simulink model "ADCS2018_Simulink_Full"  (R2018a)
settings: Solver=FixedStepAuto  StartTime=0.0  StopTime=tfinal  FixedStep=ss  RelTol=1e-3  EnableMultiTasking=on
values from neighbouring files (symbols this model uses):
  a1 = -9/11    (= -0.818181818182)    [orbitParameters.m]
  b0 = 2/11    (= 0.181818181818)    [orbitParameters.m]
  b1 = -2/11    (= -0.181818181818)    [orbitParameters.m]
  cr = 1    [orbitParameters.m]
  I = 10^-6*[29290.7 53.8 0.5; 53.8 28639.4 0; 0.5 0 5490.1]    [orbitParameters.m]
  Iw = Hw * 180 / (8000*pi)    [orbitParameters.m]
  Kd = 3.68819*1e-4*0.1/8e-11    (= 461023.75)    [orbitParameters.m]
  kd = 2e-2*min(diag(I))*0.2/3e-9    [orbitParameters.m]
  kep_init = [ semimajoraxis ... (first row only)    [orbitParameters.m]
  Kp = 3.29838*1e-8*0.1/1e-12    (= 3298.38)    [orbitParameters.m]
  mc_max = 0.2    [orbitParameters.m]
  mr = [0.001; -0.001; 0.005]    [orbitParameters.m]
  mr_max = 0.2    [orbitParameters.m]
  omega_o = sqrt(mu/abs(semimajoraxis)^3)    [orbitParameters.m]
  Pitch = 90    [orbitParameters.m]
  Roll = 0    [orbitParameters.m]
  Rx = 30    [orbitParameters.m]
  Ry = 30    [orbitParameters.m]
  Rz = 83    [orbitParameters.m]
  tme_init = [2018 06 07 16 15 0]    [orbitParameters.m]
  vc_max = 5    [orbitParameters.m]
  vr_max = 2.5    [orbitParameters.m]
  wx = 30    [orbitParameters.m]
  wy = 0    [orbitParameters.m]
  wz = 0    [orbitParameters.m]
  Yaw = 0    [orbitParameters.m]
undefined symbols (not defined in the file or in its folder): GHemb, GHsim, sigbuilder_block, SVemb, SVsim, Yemb, Ysim
libraries: My_library x27, simulink x5, vrlib x2, dspindex x1, dspmathops x1
(part 1 of 2)
settings Model: Creator=Navya  LastModifiedBy=IGOSAT
settings SolverCC: AutoInsertRateTranBlk=on
settings DataIOCC: LimitDataPoints=on
settings OptimizationCC: OptimizeBlockIOStorage=off  BufferReuse=off  GlobalBufferReuse=off  ExpressionFolding=off  LocalBlockOutputs=off  LifeSpan=inf  OptimizeDataStoreBuffers=off  BusAssignmentInplaceUpdate=off
settings DebuggingCC: AllowSymbolicDim=off  SFUnexpectedBacktrackingDiag=warning  SFNoUnconditionalDefaultTransitionDiag=warning  SFExecutionAtInitializationDiag=none
settings ModelReferenceCC: PropagateSignalLabelsOutOfModel=off
settings RTWCC: GenerateReport=on  LaunchReport=on  TargetLang=C++  CheckMdlBeforeBuild=Warning
settings CodeAppCC: StateflowObjectComments=on  MATLABSourceComments=on
settings GRTTargetCC: TargetLangStandard=C89/C90 (ANSI)  MatFileLogging=off  MultiInstanceERTCode=on  CodeInterfacePackaging=C++ class
settings ConfigComp: CovMetricSettings=dw  CovHtmlReporting=on  CovSaveCumulativeToWorkspaceVar=on  CovSaveSingleToWorkspaceVar=on  CovExternalEMLEnable=off

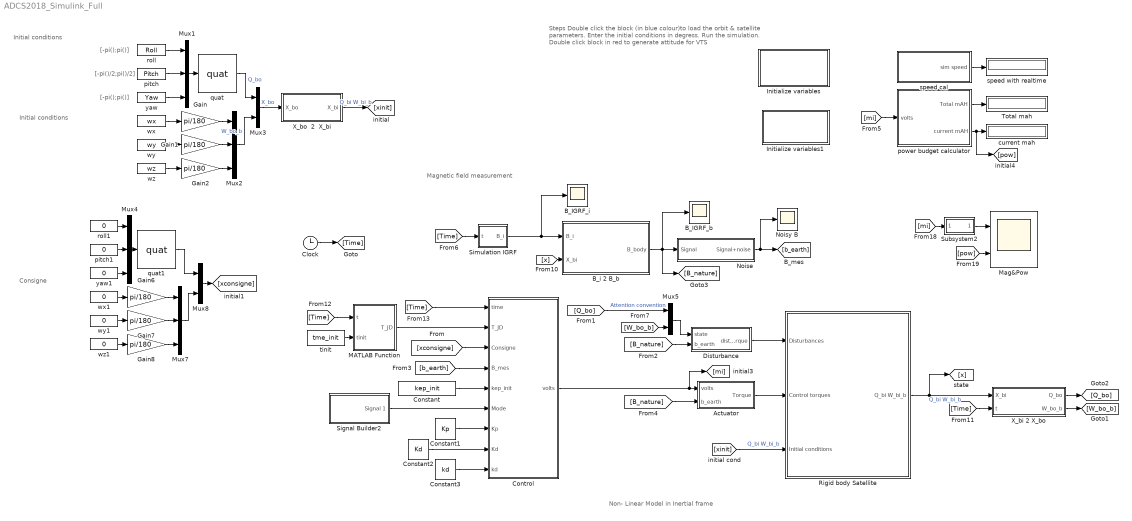
== system ADCS2018_Simulink_Full ==
  note: Magnetic field measurement
  note: [-pi();pi()]
  note: [-pi()/2;pi()/2]
  note: Initial conditions
  note: Non- Linear Model in Inertial frame
  note: Initial conditions
  note: Steps
      |
      | Double click the block (in blue colour)to load the orbit & satellite parameters.
      |
      | Enter the initial conditions in degress.
      |
      | Run the simulation.
      |
      | Double click block in red to generate
      | attitude for VTS
  note: Consigne
  note: [-pi();pi()]
  Actuator : Subsystem  TreatAsAtomicUnit=on  SystemSampleTime=ss
  B_IGRF_b : Scope
  B_IGRF_i : Scope
  B_i 2 B_b : Subsystem
  Clock : Clock
  Constant : Constant  Value=kep_init
  Constant1 : Constant  Value=Kp
  Constant2 : Constant  Value=Kd
  Constant3 : Constant  Value=kd
  Control : Subsystem  TreatAsAtomicUnit=on  SystemSampleTime=cr  RTWFcnName=Controller
      settings: RTWSystemCode=Nonreusable function  RTWFcnNameOpts=User specified  RTWFileNameOpts=Use function name
  Disturbance : Subsystem
  Gain{,1..2,6..8} (6 alike) : Gain  Gain=pi/180
  Initialize variables : Subsystem
      settings: OpenFcn=orbitParameters
      mask Display: disp('Double Click\n to Initialize orbit')
  Initialize variables1 : Subsystem
      settings: OpenFcn=toVTS
      mask Display: disp('Double Click\n to generate \n attitude for VTS')
  MATLAB Function : MATLAB Function  TreatAsAtomicUnit=on
  Mag&Pow : Scope  NumInputPorts=2
  Mux{1..2,4,7} (4 alike) : Mux  Inputs=3
  Mux3 : Mux  Inputs=2
  Mux5 : Mux  Inputs=2
  Mux8 : Mux  Inputs=2
  Noise : Subsystem
  Noisy B : Scope
  Rigid body Satellite : Subsystem  mask{I=I, wo=omega_o}
      mask prompts: I "Inertia"; wo "Orbit Velocity"
      mask Display:
      | image(imread('download.jpg'))
      | port_label('input',1,'disturbances')
      | port_label('input',2,'Control torques')
      | port_label('input',3,'Initial conditions')
      | port_label('output',1,'[q_bo;w_bo]')
  Signal Builder2 : Subsystem  Tag=STV Subsys  LoadFcn=sigbuilder_block('load');  StartFcn=sigbuilder_block('start');  StopFcn=sigbuilder_block('stop');  ClipboardFcn=sigbuilder_block('clipboard');  mask(Sigbuilder block){tuvar=[0:10]}
      mask help: Simulink:masks:SigbuilderBlock_MD
      mask init:
      | if ~strcmp(get_param(bdroot(gcbh),'SimulationStatus'),'stopped') tuvar = sigbuilder_block('maskInit'); end
      settings: CopyFcn=sigbuilder_block('copy');  DeleteFcn=sigbuilder_block('delete');  ModelCloseFcn=sigbuilder_block('modelClose');  PreSaveFcn=sigbuilder_block('preSave');  PauseFcn=sigbuilder_block('pause');  ContinueFcn=sigbuilder_block('continue');  NameChangeFcn=sigbuilder_block('namechange');  OpenFcn=sigbuilder_block('open',[370.5 320.25 551.25 282 ]);  CloseFcn=sigbuilder_block('close');
      mask Display: plot(0, 0, 100, 100,[2, 2, 32, 32, 2], [68, 8, 8, 68, 68],[32, 2], [38, 38], [32, 19, 2],[53, 60, 44], [32, 17, 17, 2],[16, 16, 31, 31]);txt = getActiveGroup(gcbh);text(2, 100, txt,'verticalAlignment', 'top');
  Simulation IGRF : Subsystem
  Subsystem2 : Subsystem
  Total mah : Display
  "X_bi 2 X_bo " : Subsystem
  X_bo  2  X_bi : Subsystem
  current mah : Display
  pitch : Constant  Value=Pitch
  pitch1 : Constant  Value=0
  power budget calculator : Subsystem
  quat : My_library/quat
      settings: SourceProductName=My Library
  quat1 : My_library/quat
      settings: SourceProductName=My Library
  roll : Constant  Value=Roll
  roll1 : Constant  Value=0
  speed cal : Subsystem
  speed with realtime : Display
  tinit : Constant  Value=tme_init
  wx : Constant  Value=wx
  wx1 : Constant  Value=0
  wy : Constant  Value=wy
  wy1 : Constant  Value=0
  wz : Constant  Value=wz
  wz1 : Constant  Value=0
  yaw : Constant  Value=Yaw
  yaw1 : Constant  Value=0
  wires:
  Disturbance/1(dist torque) -> Rigid body Satellite/1(Disturbances)
  Mux5/1 -> Disturbance/1(state)
  Gain1/1 -> Mux2/2
  Gain2/1 -> Mux2/3
  wz/1 -> Gain2/1
  Mux2/1 -> Mux3/2  "W_bo_b"
  wx/1 -> Gain/1
  quat/1 -> Mux3/1  "Q_bo"
  Gain/1 -> Mux2/1
  wy/1 -> Gain1/1
  Mux1/1 -> quat/1
  roll/1 -> Mux1/1
  pitch/1 -> Mux1/2
  yaw/1 -> Mux1/3
  [xinit] -> Rigid body Satellite/3(Initial conditions)  "Q_bi W_bi_b"
  Actuator/1(Torque) -> Rigid body Satellite/2(Control torques)
  Rigid body Satellite/1(Q_bi W_bi_b) -> "X_bi 2 X_bo "/1(X_bi), [x]  "Q_bi W_bi_b"
  power budget calculator/2(current mAH) -> [pow], current mah/1
  power budget calculator/1(Total mAH) -> Total mah/1
  speed cal/1(sim speed) -> speed with realtime/1
  "X_bi 2 X_bo "/2(W_bo_b) -> [W_bo_b]
  [mi] -> power budget calculator/1(volts)
  [B_nature] -> Actuator/2(b_earth)
  [B_nature] -> Disturbance/2(b_earth)
  Simulation IGRF/1(B_i) -> B_IGRF_i/1, B_i 2 B_b/1("B_i ")
  [x] -> B_i 2 B_b/2(X_bi)
  Gain7/1 -> Mux7/2
  Gain8/1 -> Mux7/3
  wz1/1 -> Gain8/1
  Mux8/1 -> [xconsigne]
  Mux7/1 -> Mux8/2
  wx1/1 -> Gain6/1
  quat1/1 -> Mux8/1
  Gain6/1 -> Mux7/1
  wy1/1 -> Gain7/1
  Mux4/1 -> quat1/1
  roll1/1 -> Mux4/1
  pitch1/1 -> Mux4/2
  yaw1/1 -> Mux4/3
  tinit/1 -> MATLAB Function/2(tinit)
  Mux3/1 -> X_bo  2  X_bi/1(X_bo)  "X_bo"
  X_bo  2  X_bi/1(X_bi) -> [xinit]  "Q_bi W_bi_b"
  Clock/1 -> [Time]
  [Time] -> MATLAB Function/1(t)
  [Time] -> "X_bi 2 X_bo "/2(t)
  "X_bi 2 X_bo "/1(Q_bo) -> [Q_bo]
  [Time] -> Simulation IGRF/1(t)
  [Q_bo] -> Mux5/1  "Attention convention"
  [W_bo_b] -> Mux5/2
  [mi] -> Subsystem2/1(In1)
  Subsystem2/1(Out1) -> Mag&Pow/1
  [pow] -> Mag&Pow/2
  B_i 2 B_b/1(B_body) -> [B_nature], B_IGRF_b/1, Noise/1(Signal)
  Noise/1(Signal+noise) -> [b_earth], Noisy B/1
  Control/1(volts) -> Actuator/1(volts), [mi]
  [Time] -> Control/1(time)
  MATLAB Function/1(T_JD) -> Control/2(T_JD)
  [xconsigne] -> Control/3(Consigne)
  [b_earth] -> Control/4(B_mes)
  Constant/1 -> Control/5(kep_init)
  Signal Builder2/1(Signal 1) -> Control/6("Mode ")
  Constant1/1 -> Control/7(Kp)
  Constant2/1 -> Control/8(Kd)
  Constant3/1 -> Control/9(kd)

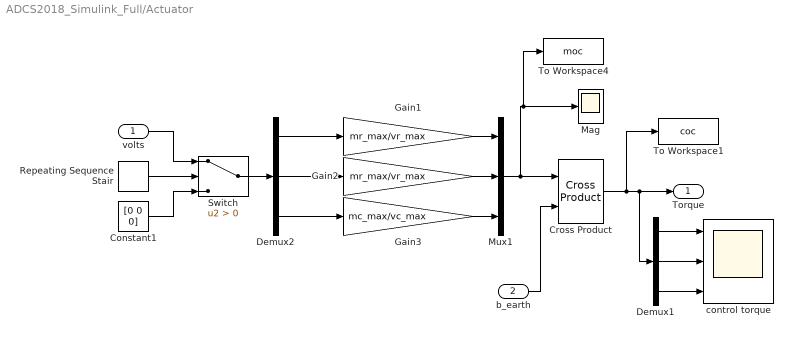
== system ADCS2018_Simulink_Full/Actuator ==
  volts : Inport
  b_earth : Inport  Port=2
  Constant1 : Constant  Value=[0 0 0]
  Cross Product : vrlib/Utilities/Cross Product
      settings: SourceProductBaseCode=VR
  Demux1 : Demux  Outputs=3
  Demux2 : Demux  Outputs=3
  Gain1 : Gain  Gain=mr_max/vr_max
  Gain2 : Gain  Gain=mr_max/vr_max
  Gain3 : Gain  Gain=mc_max/vc_max
  Mag : Scope
  Mux1 : Mux  Inputs=3
  Repeating Sequence Stair : simulink/Sources/Repeating Sequence Stair  OutValues=[1 1 1 1 1 1 1 0 0 0]  tsamp=-1  OutMin=[]  OutMax=[]  OutDataTypeStr=double  OutputDataTypeScalingMode=double  OutDataType=fixdt(0,8)  ConRadixGroup=Best Precision: Vector-wise  OutScaling=2^-12
  Switch : Switch  Criteria=u2 > Threshold
  To Workspace1 : ToWorkspace  VariableName=coc  SampleTime=-1
  To Workspace4 : ToWorkspace  VariableName=moc  SampleTime=-1
  control torque : Scope  NumInputPorts=3
  Torque : Outport
  wires:
  Demux1/1 -> control torque/1
  Demux1/2 -> control torque/2
  Demux1/3 -> control torque/3
  Gain1/1 -> Mux1/1
  Gain2/1 -> Mux1/2
  Gain3/1 -> Mux1/3
  Demux2/1 -> Gain1/1
  Demux2/2 -> Gain2/1
  Demux2/3 -> Gain3/1
  Mux1/1 -> To Workspace4/1, Mag/1, Cross Product/1
  Cross Product/1 -> To Workspace1/1, Torque/1, Demux1/1
  b_earth/1 -> Cross Product/2
  Repeating Sequence Stair/1 -> Switch/2
  Constant1/1 -> Switch/3
  volts/1 -> Switch/1
  Switch/1 -> Demux2/1

== system ADCS2018_Simulink_Full/B_i 2 B_b ==
  "B_i " : Inport  PortDimensions=3
  X_bi : Inport  Port=2
  Constant : Constant  Value=0
  Demux : Demux
  Demux1 : Demux  Outputs=7
  Mux : Mux
  Mux1 : Mux  Inputs=2
  Mux2 : Mux  Inputs=3
  Mux5 : Mux  Inputs=3
  No need for the angular velocity : Terminator
  Terminator : Terminator
  quat multiply1 : My_library/quat multiply
      settings: SourceProductName=My Library
  quat multiply2 : My_library/quat multiply
      settings: SourceProductName=My Library
  quaternion conjugate : My_library/quaternion conjugate
      settings: SourceProductName=My Library
  B_body : Outport  PortDimensions=3
  wires:
  X_bi/1 -> Demux1/1
  Demux1/5 -> Mux5/1
  Demux1/6 -> Mux5/2
  Demux1/7 -> Mux5/3
  Mux5/1 -> No need for the angular velocity/1
  Demux1/1 -> Mux/1
  Demux1/2 -> Mux/2
  Demux1/3 -> Mux/3
  Demux1/4 -> Mux/4
  Mux/1 -> quat multiply1/2, quaternion conjugate/1
  "B_i "/1 -> Mux1/2
  quaternion conjugate/1 -> quat multiply2/1
  Constant/1 -> Mux1/1
  Mux1/1 -> quat multiply2/2
  quat multiply2/1 -> quat multiply1/1
  quat multiply1/1 -> Demux/1
  Demux/2 -> Mux2/1
  Demux/3 -> Mux2/2
  Demux/4 -> Mux2/3
  Mux2/1 -> B_body/1
  Demux/1 -> Terminator/1

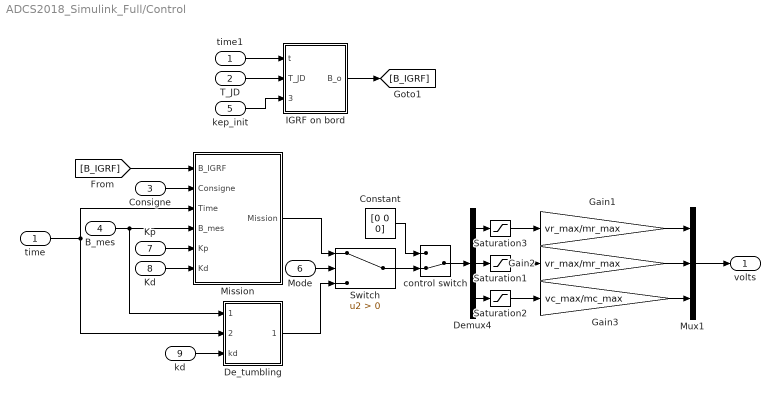
== system ADCS2018_Simulink_Full/Control ==
  time : Inport
  T_JD : Inport  Port=2
  Consigne : Inport  Port=3  PortDimensions=7
  B_mes : Inport  Port=4  PortDimensions=3
  kep_init : Inport  Port=5
  "Mode " : Inport  Port=6
  Kp : Inport  Port=7  PortDimensions=1
  Kd : Inport  Port=8  PortDimensions=1
  kd : Inport  Port=9  PortDimensions=1
  Constant : Constant  Value=[0 0 0]
  De_tumbling : Subsystem
  Demux4 : Demux  Outputs=3
  Gain1 : Gain  Gain=vr_max/mr_max
  Gain2 : Gain  Gain=vr_max/mr_max
  Gain3 : Gain  Gain=vc_max/mc_max
  IGRF on bord : Subsystem
  Mission : Subsystem
  Mux1 : Mux  Inputs=3
  Saturation1 : Saturate  UpperLimit=mr_max  LowerLimit=-mr_max
  Saturation2 : Saturate  UpperLimit=mc_max  LowerLimit=-mc_max
  Saturation3 : Saturate  UpperLimit=mr_max  LowerLimit=-mr_max
  Switch : Switch  Criteria=u2 > Threshold
  control switch : ManualSwitch  CurrentSetting=0
  time1 : InportShadow
  volts : Outport  PortDimensions=3
  wires:
  Demux4/3 -> Saturation2/1
  Demux4/2 -> Saturation1/1
  Demux4/1 -> Saturation3/1
  Saturation3/1 -> Gain1/1
  Gain1/1 -> Mux1/1
  Saturation2/1 -> Gain3/1
  Gain2/1 -> Mux1/2
  Saturation1/1 -> Gain2/1
  Gain3/1 -> Mux1/3
  control switch/1 -> Demux4/1
  Constant/1 -> control switch/1
  time/1 -> De_tumbling/2(Time), Mission/3(Time)
  Consigne/1 -> Mission/2(Consigne)
  [B_IGRF] -> Mission/1(B_IGRF)
  time1/1 -> IGRF on bord/1(t)
  IGRF on bord/1(B_o) -> [B_IGRF]
  T_JD/1 -> IGRF on bord/2(T_JD)
  "Mode "/1 -> Switch/2
  B_mes/1 -> De_tumbling/1(B_mes), Mission/4(B_mes)
  Mission/1(Mission) -> Switch/1
  De_tumbling/1(B_dot) -> Switch/3
  Switch/1 -> control switch/2
  Mux1/1 -> volts/1
  kep_init/1 -> IGRF on bord/3(kep_init)
  Kp/1 -> Mission/5(Kp)
  Kd/1 -> Mission/6(Kd)
  kd/1 -> De_tumbling/3(kd)

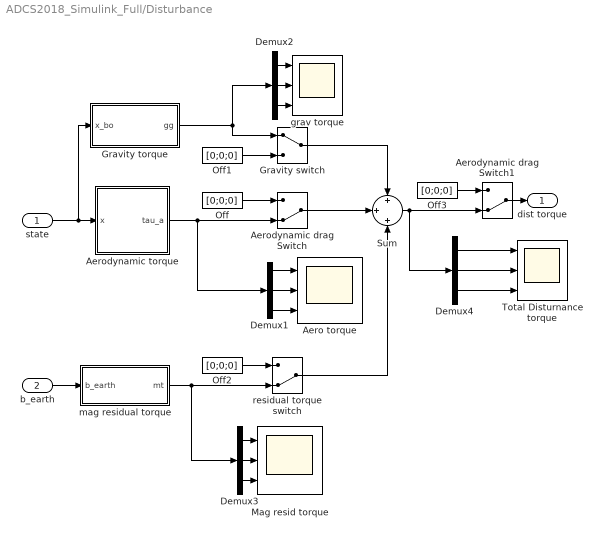
== system ADCS2018_Simulink_Full/Disturbance ==
  state : Inport
  b_earth : Inport  Port=2
  Aero torque : Scope  NumInputPorts=3
  Aerodynamic drag Switch : ManualSwitch  CurrentSetting=0
  Aerodynamic drag Switch1 : ManualSwitch  CurrentSetting=0
  Aerodynamic torque : MATLAB Function  TreatAsAtomicUnit=on
  Demux{1..4} (4 alike) : Demux  Outputs=3
  Gravity switch : ManualSwitch
  Gravity torque : Subsystem  mask{I=I, wo=omega_o}
      mask prompts: I "Inertia"; wo "orbit rate"
  Mag resid torque : Scope  NumInputPorts=3
  Off{,1..3} (4 alike) : Constant  Value=[0;0;0]
  Sum : Sum  Inputs=+|+|+
  Total Disturnance torque : Scope  NumInputPorts=3
  grav torque : Scope  NumInputPorts=3
  mag residual torque : Subsystem
  residual torque switch : ManualSwitch  CurrentSetting=0
  dist torque : Outport  PortDimensions=3
  wires:
  Gravity switch/1 -> Sum/1
  state/1 -> Gravity torque/1(x_bo), Aerodynamic torque/1(x)
  Aerodynamic drag Switch/1 -> Sum/2
  residual torque switch/1 -> Sum/3
  Aerodynamic torque/1(tau_a) -> Demux1/1, Aerodynamic drag Switch/2
  Gravity torque/1(gg) -> Gravity switch/1, Demux2/1
  Demux1/1 -> Aero torque/1
  Demux1/2 -> Aero torque/2
  Demux1/3 -> Aero torque/3
  mag residual torque/1(mt) -> Demux3/1, residual torque switch/2
  Demux3/1 -> Mag resid torque/1
  Demux3/2 -> Mag resid torque/2
  Demux3/3 -> Mag resid torque/3
  Sum/1 -> Aerodynamic drag Switch1/2, Demux4/1
  Demux4/1 -> Total Disturnance torque/1
  Demux4/2 -> Total Disturnance torque/2
  Demux4/3 -> Total Disturnance torque/3
  Off/1 -> Aerodynamic drag Switch/1
  b_earth/1 -> mag residual torque/1(b_earth)
  Off1/1 -> Gravity switch/2
  Demux2/1 -> grav torque/1
  Demux2/2 -> grav torque/2
  Demux2/3 -> grav torque/3
  Off2/1 -> residual torque switch/1
  Off3/1 -> Aerodynamic drag Switch1/1
  Aerodynamic drag Switch1/1 -> dist torque/1

== system ADCS2018_Simulink_Full/Initialize variables ==

== system ADCS2018_Simulink_Full/Initialize variables1 ==

== system ADCS2018_Simulink_Full/Noise ==
  Signal : Inport
  Add : Sum
  Band-Limited White Noise1 : simulink/Sources/Band-Limited White Noise  Cov=mn  Ts=2  seed=[14305]
  Band-Limited White Noise2 : simulink/Sources/Band-Limited White Noise  Cov=mn  Ts=2  seed=[23341]
  Band-Limited White Noise3 : simulink/Sources/Band-Limited White Noise  Cov=mn  Ts=2  seed=[23582]
  Mux3 : Mux  Inputs=3
  Signal+noise : Outport
  wires:
  Band-Limited White Noise2/1 -> Mux3/2
  Band-Limited White Noise3/1 -> Mux3/3
  Add/1 -> Signal+noise/1
  Signal/1 -> Add/1
  Band-Limited White Noise1/1 -> Mux3/1
  Mux3/1 -> Add/2

== system ADCS2018_Simulink_Full/Rigid body Satellite ==
  Disturbances : Inport  PortDimensions=3
  Control torques : Inport  Port=2
  Initial conditions : Inport  Port=3
  Demux : Demux  Outputs=7
  Dynamics : Subsystem
  Kinematics : Subsystem
  Mux : Mux  Inputs=2
  Mux1 : Mux
  Mux2 : Mux  Inputs=3
  Q_bi W_bi_b : Outport  PortDimensions=7
  wires:
  Disturbances/1 -> Dynamics/2(disturbances)
  Control torques/1 -> Dynamics/1(Control torques)
  Dynamics/1(W_bi_b) -> Kinematics/1(W_bi_b), Mux/2
  Mux/1 -> Q_bi W_bi_b/1
  Initial conditions/1 -> Demux/1  "Q_bi W_bi_b"
  Demux/1 -> Mux1/1
  Demux/2 -> Mux1/2
  Demux/3 -> Mux1/3
  Demux/4 -> Mux1/4
  Demux/6 -> Mux2/2
  Demux/5 -> Mux2/1
  Demux/7 -> Mux2/3
  Mux1/1 -> [qinit]
  [qinit] -> Kinematics/2(Init quat)  "Q_bi"
  Mux2/1 -> [winit]
  [winit] -> Dynamics/3(Initial rate)  "W_bi_b"
  Kinematics/1(Q_bi) -> Mux/1

== system ADCS2018_Simulink_Full/Signal Builder2 ==
  Demux : Demux  Tag=STV Demux  Outputs=1
  FromWs : FromWorkspace  Tag=STV FromWs  VariableName=tuvar  SampleTime=0
      SigBuilderData=|
      | common.afterFinalStr = 'Extrapolate'
      | common.sampleTime = 0
      | dataSet.timeRange = [0 146369.116664]
      | dataSet.name = 'Group 1'
      | sbobj.Groups.Name = 'Group 1'
      | sbobj.Groups.Signals.Name = 'Signal 1'
      | sbobj.Groups.Signals.XData = [0 40000 40000 146369.116664]
      | sbobj.Groups.Signals.YData = [0 0 1 1]
      | sbobj.Groups.TimeRange = [0 146369.116664]
  Signal 1 : Outport  Tag=STV Outport
  wires:
  FromWs/1 -> Demux/1
  Demux/1 -> Signal 1/1

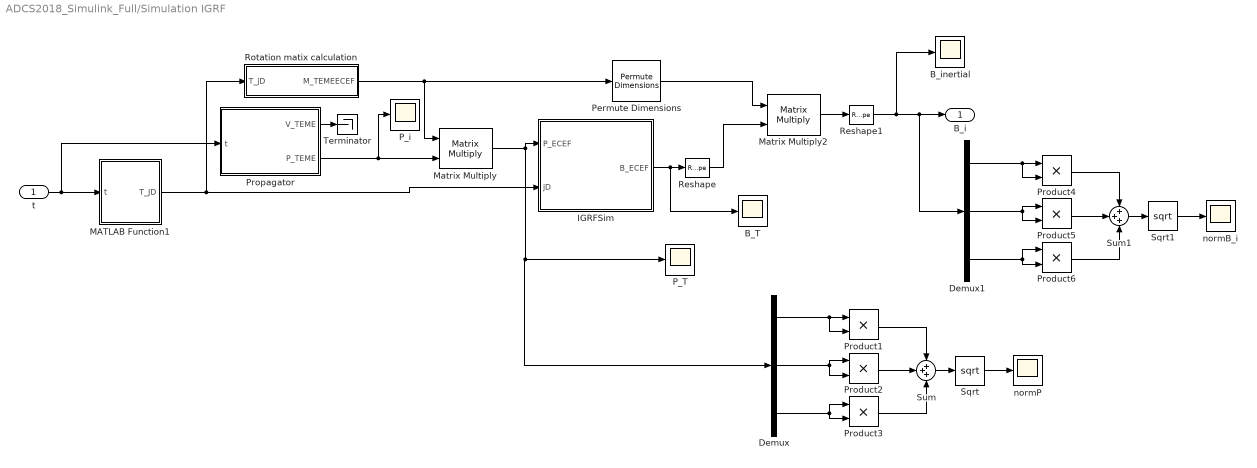
== system ADCS2018_Simulink_Full/Simulation IGRF ==
  t : Inport
  B_T : Scope
  B_inertial : Scope
  Demux : Demux  Outputs=3
  Demux1 : Demux  Outputs=3
  IGRFSim : MATLAB Function  TreatAsAtomicUnit=on
  MATLAB Function1 : MATLAB Function  TreatAsAtomicUnit=on
  Matrix Multiply : Product  Multiplication=Matrix(*)
  Matrix Multiply2 : Product  Multiplication=Matrix(*)
  P_T : Scope
  P_i : Scope
  Permute Dimensions : PermuteDimensions
  Product{1..6} (6 alike) : Product
  Propagator : MATLAB Function  TreatAsAtomicUnit=on
  Reshape : Reshape  OutputDimensionality=Column vector (2-D)
  Reshape1 : Reshape
  Rotation matix calculation : Subsystem
  Sqrt : Sqrt  SaturateOnIntegerOverflow=on
  Sqrt1 : Sqrt  SaturateOnIntegerOverflow=on
  Sum : Sum  Inputs=3
  Sum1 : Sum  Inputs=3
  Terminator : Terminator
  normB_i : Scope
  normP : Scope
  B_i : Outport
  wires:
  Rotation matix calculation/1(M_TEMEECEF) -> Permute Dimensions/1, Matrix Multiply/1
  IGRFSim/1(B_ECEF) -> B_T/1, Reshape/1
  Reshape/1 -> Matrix Multiply2/2
  MATLAB Function1/1(T_JD) -> Rotation matix calculation/1(T_jD), IGRFSim/2(jD)
  Matrix Multiply2/1 -> Reshape1/1
  t/1 -> Propagator/1(t), MATLAB Function1/1(t)
  Reshape1/1 -> B_inertial/1, Demux1/1, B_i/1
  Propagator/1(V_TEME) -> Terminator/1
  Permute Dimensions/1 -> Matrix Multiply2/1
  Demux/3 -> Product3/2, Product3/1
  Matrix Multiply/1 -> P_T/1, Demux/1, IGRFSim/1(P_ECEF)
  Sum/1 -> Sqrt/1
  Product1/1 -> Sum/1
  Demux/1 -> Product1/2, Product1/1
  Product2/1 -> Sum/2
  Demux/2 -> Product2/2, Product2/1
  Product3/1 -> Sum/3
  Sqrt/1 -> normP/1
  Propagator/2(P_TEME) -> Matrix Multiply/2, P_i/1
  Sqrt1/1 -> normB_i/1
  Product5/1 -> Sum1/2
  Product6/1 -> Sum1/3
  Demux1/1 -> Product4/2, Product4/1
  Demux1/2 -> Product5/2, Product5/1
  Product4/1 -> Sum1/1
  Demux1/3 -> Product6/2, Product6/1
  Sum1/1 -> Sqrt1/1

== system ADCS2018_Simulink_Full/Subsystem2 ==
  In1 : Inport
  Demux3 : Demux  Outputs=3
  Gain6 : Gain  Gain=mr_max/vr_max
  Gain7 : Gain  Gain=mr_max/vr_max
  Gain8 : Gain  Gain=mc_max/vc_max
  Mux7 : Mux  Inputs=3
  Out1 : Outport
  wires:
  Gain7/1 -> Mux7/2
  Demux3/2 -> Gain7/1
  Mux7/1 -> Out1/1
  Demux3/1 -> Gain6/1
  Gain6/1 -> Mux7/1
  Gain8/1 -> Mux7/3
  In1/1 -> Demux3/1
  Demux3/3 -> Gain8/1

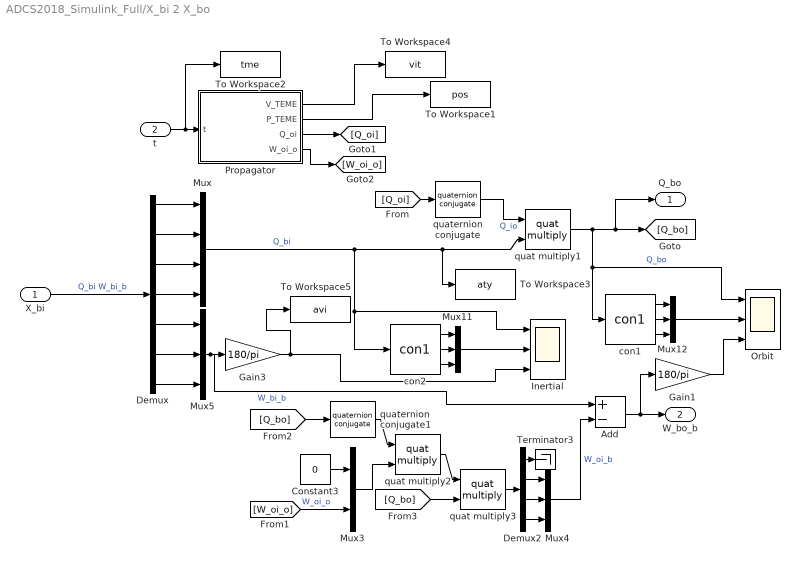
== system ADCS2018_Simulink_Full/X_bi 2 X_bo  ==
  X_bi : Inport
  t : Inport  Port=2
  Add : Sum  Inputs=+-
  Constant3 : Constant  Value=0
  Demux : Demux  Outputs=7
  Demux2 : Demux
  Gain1 : Gain  Gain=180/pi
  Gain3 : Gain  Gain=180/pi
  Inertial : Scope  NumInputPorts=3
  Mux : Mux
  Mux{4..5,11..12} (4 alike) : Mux  Inputs=3
  Mux3 : Mux  Inputs=2
  Orbit : Scope  NumInputPorts=3
  Propagator : MATLAB Function  TreatAsAtomicUnit=on
  Terminator3 : Terminator
  To Workspace1 : ToWorkspace  VariableName=pos  SampleTime=-1
  To Workspace2 : ToWorkspace  VariableName=tme  SampleTime=-1
  To Workspace3 : ToWorkspace  VariableName=aty  SampleTime=-1
  To Workspace4 : ToWorkspace  VariableName=vit  SampleTime=-1
  To Workspace5 : ToWorkspace  VariableName=avi  SampleTime=-1
  con1 : My_library/con1
      settings: SourceProductName=My Library
  con2 : My_library/con1
      settings: SourceProductName=My Library
  quat multiply1 : My_library/quat multiply
      settings: SourceProductName=My Library
  quat multiply2 : My_library/quat multiply
      settings: SourceProductName=My Library
  quat multiply3 : My_library/quat multiply
      settings: SourceProductName=My Library
  quaternion conjugate : My_library/quaternion conjugate
      settings: SourceProductName=My Library
  quaternion conjugate1 : My_library/quaternion conjugate
      settings: SourceProductName=My Library
  Q_bo : Outport
  W_bo_b : Outport  Port=2
  wires:
  X_bi/1 -> Demux/1  "Q_bi W_bi_b"
  Demux/5 -> Mux5/1
  Demux/6 -> Mux5/2
  Demux/7 -> Mux5/3
  Demux/1 -> Mux/1
  Demux/2 -> Mux/2
  Demux/3 -> Mux/3
  Demux/4 -> Mux/4
  Mux/1 -> con2/1, Inertial/1, To Workspace3/1, quat multiply1/2  "Q_bi"
  Propagator/1(V_TEME) -> To Workspace4/1
  t/1 -> To Workspace2/1, Propagator/1(t)
  quaternion conjugate/1 -> quat multiply1/1  "Q_io"
  quat multiply1/1 -> Q_bo/1, [Q_bo], Orbit/1, con1/1  "Q_bo"
  Constant3/1 -> Mux3/1
  Demux2/3 -> Mux4/2
  quat multiply3/1 -> Demux2/1
  [Q_bo] -> quat multiply3/2
  [W_oi_o] -> Mux3/2  "W_oi_o"
  quat multiply2/1 -> quat multiply3/1
  [Q_bo] -> quaternion conjugate1/1
  Mux3/1 -> quat multiply2/2
  Demux2/4 -> Mux4/3
  Demux2/1 -> Terminator3/1
  quaternion conjugate1/1 -> quat multiply2/1
  Mux4/1 -> Add/2  "W_oi_b"
  Demux2/2 -> Mux4/1
  Mux5/1 -> Add/1, Gain3/1  "W_bi_b"
  Add/1 -> W_bo_b/1, Gain1/1
  Gain3/1 -> Inertial/3, To Workspace5/1
  con2/2 -> Mux11/2
  con2/3 -> Mux11/3
  con2/1 -> Mux11/1
  Mux11/1 -> Inertial/2
  con1/1 -> Mux12/1
  con1/3 -> Mux12/3
  con1/2 -> Mux12/2
  Gain1/1 -> Orbit/3
  Mux12/1 -> Orbit/2
  Propagator/2(P_TEME) -> To Workspace1/1
  Propagator/3(Q_oi) -> [Q_oi]
  [Q_oi] -> quaternion conjugate/1
  Propagator/4(W_oi_o) -> [W_oi_o]

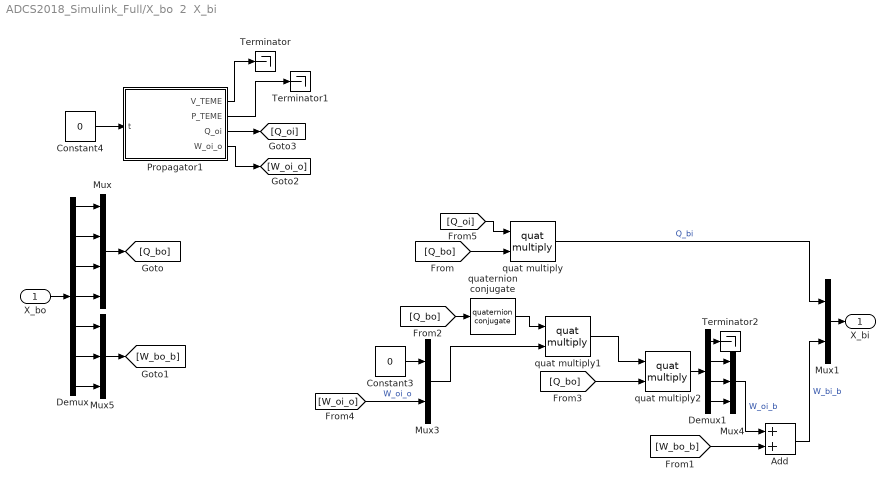
== system ADCS2018_Simulink_Full/X_bo  2  X_bi ==
  X_bo : Inport
  Add : Sum
  Constant3 : Constant  Value=0
  Constant4 : Constant  Value=0
  Demux : Demux  Outputs=7
  Demux1 : Demux
  Mux : Mux
  Mux1 : Mux  Inputs=2
  Mux3 : Mux  Inputs=2
  Mux4 : Mux  Inputs=3
  Mux5 : Mux  Inputs=3
  Propagator1 : MATLAB Function  TreatAsAtomicUnit=on
  Terminator : Terminator
  Terminator1 : Terminator
  Terminator2 : Terminator
  quat multiply : My_library/quat multiply
      settings: SourceProductName=My Library
  quat multiply1 : My_library/quat multiply
      settings: SourceProductName=My Library
  quat multiply2 : My_library/quat multiply
      settings: SourceProductName=My Library
  quaternion conjugate : My_library/quaternion conjugate
      settings: SourceProductName=My Library
  X_bi : Outport
  wires:
  X_bo/1 -> Demux/1
  Demux/1 -> Mux/1
  Demux/2 -> Mux/2
  Demux/3 -> Mux/3
  Demux/4 -> Mux/4
  Demux/5 -> Mux5/1
  Demux/6 -> Mux5/2
  Demux/7 -> Mux5/3
  Mux5/1 -> [W_bo_b]
  Propagator1/1(V_TEME) -> Terminator/1
  [Q_bo] -> quat multiply/2
  Propagator1/2(P_TEME) -> Terminator1/1
  Mux1/1 -> X_bi/1
  quat multiply/1 -> Mux1/1  "Q_bi"
  [Q_bo] -> quaternion conjugate/1
  [W_oi_o] -> Mux3/2  "W_oi_o"
  Mux3/1 -> quat multiply1/2
  Constant3/1 -> Mux3/1
  quaternion conjugate/1 -> quat multiply1/1
  quat multiply1/1 -> quat multiply2/1
  [Q_bo] -> quat multiply2/2
  quat multiply2/1 -> Demux1/1
  Demux1/2 -> Mux4/1
  Demux1/3 -> Mux4/2
  Demux1/4 -> Mux4/3
  Mux4/1 -> Add/1  "W_oi_b"
  [W_bo_b] -> Add/2
  Demux1/1 -> Terminator2/1
  Add/1 -> Mux1/2  "W_bi_b"
  Mux/1 -> [Q_bo]
  Constant4/1 -> Propagator1/1(t)
  Propagator1/4(W_oi_o) -> [W_oi_o]
  Propagator1/3(Q_oi) -> [Q_oi]
  [Q_oi] -> quat multiply/1

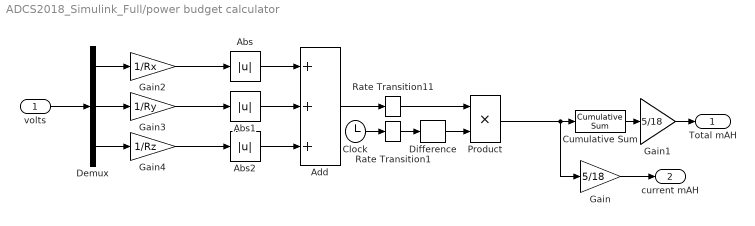
== system ADCS2018_Simulink_Full/power budget calculator ==
  volts : Inport
  Abs : Abs
  Abs1 : Abs
  Abs2 : Abs
  Add : Sum  Inputs=+++
  Clock : Clock
  Cumulative Sum : dspmathops/Cumulative Sum  dim=Channels (running sum)  InputProcessing=Columns as channels (frame based)  reset_popup=None  roundingMode=Floor  overflowMode=off  outputDataTypeStr=Inherit: Same as accumulator  outputMin=[]  outputMax=[]  outputLastDataTypeStr=Inherit: Same as accumulator
      settings: SourceProductName=DSP System Toolbox
  Demux : Demux  Outputs=3
  Difference : simulink/Discrete/Difference  ICPrevInput=0.0  InputProcessing=Inherited  OutMin=[]  OutMax=[]  OutDataType=fixdt(1, 16)  OutScaling=2^-10  DoSatur=off
  Gain : Gain  Gain=5/18
  Gain1 : Gain  Gain=5/18
  Gain2 : Gain  Gain=1/Rx
  Gain3 : Gain  Gain=1/Ry
  Gain4 : Gain  Gain=1/Rz
  Product : Product
  Rate Transition1 : RateTransition
  Rate Transition11 : RateTransition
  Total mAH : Outport
  current mAH : Outport  Port=2
  wires:
  Add/1 -> Rate Transition11/1
  Abs/1 -> Add/1
  Abs1/1 -> Add/2
  Abs2/1 -> Add/3
  Demux/3 -> Gain4/1
  Demux/2 -> Gain3/1
  Demux/1 -> Gain2/1
  volts/1 -> Demux/1
  Rate Transition11/1 -> Product/1
  Rate Transition1/1 -> Difference/1
  Difference/1 -> Product/2
  Clock/1 -> Rate Transition1/1
  Product/1 -> Gain/1, Cumulative Sum/1
  Cumulative Sum/1 -> Gain1/1
  Gain1/1 -> Total mAH/1
  Gain/1 -> current mAH/1
  Gain2/1 -> Abs/1
  Gain4/1 -> Abs2/1
  Gain3/1 -> Abs1/1

== system ADCS2018_Simulink_Full/speed cal ==
  Clock1 : Clock
  MATLAB Function : MATLAB Function  TreatAsAtomicUnit=on
  sim speed : Outport
  wires:
  MATLAB Function/1(y) -> sim speed/1
  Clock1/1 -> MATLAB Function/1(u)

== system ADCS2018_Simulink_Full/Control/De_tumbling ==
  B_mes : Inport
  Time : Inport  Port=2
  kd : Inport  Port=3
  Add : Sum  Inputs=-+
  Add7 : Sum  Inputs=+-
  Divide2 : Product  Inputs=**/
  Unit Delay : UnitDelay  SampleTime=-1
  Unit Delay1 : UnitDelay  InitialCondition=-1  SampleTime=-1
  B_dot : Outport
  wires:
  B_mes/1 -> Unit Delay/1, Add/1
  Unit Delay/1 -> Add/2
  Unit Delay1/1 -> Add7/2
  Add/1 -> Divide2/1
  Time/1 -> Unit Delay1/1, Add7/1
  Divide2/1 -> B_dot/1
  Add7/1 -> Divide2/3
  kd/1 -> Divide2/2

== system ADCS2018_Simulink_Full/Control/IGRF on bord ==
  t : Inport
  T_JD : Inport  Port=2
  kep_init : Inport  Port=3
  Frame change2 : Subsystem
  IGRFEmb : MATLAB Function  TreatAsAtomicUnit=on
  Matrix Multiply : Product  Multiplication=Matrix(*)
  Matrix Multiply2 : Product  Multiplication=Matrix(*)
  Permute Dimensions : PermuteDimensions
  Propagator : MATLAB Function  TreatAsAtomicUnit=on
  Reshape : Reshape  OutputDimensionality=Column vector (2-D)
  Reshape1 : Reshape
  Rotation matix calculation : Subsystem
  Terminator : Terminator
  quaternion conjugate2 : My_library/quaternion conjugate
      settings: SourceProductName=My Library
  B_o : Outport
  wires:
  Matrix Multiply/1 -> IGRFEmb/1(P_ECEF)
  Rotation matix calculation/1(M_TEMEECEF) -> Matrix Multiply/1, Permute Dimensions/1
  IGRFEmb/1(B_ECEF) -> Reshape/1
  Reshape/1 -> Matrix Multiply2/2
  Matrix Multiply2/1 -> Reshape1/1
  t/1 -> Propagator/1(t)
  Propagator/1(V_TEME) -> Terminator/1
  Permute Dimensions/1 -> Matrix Multiply2/1
  Propagator/3(Q_oi) -> [Q_oi]
  Frame change2/1("V[2] ") -> B_o/1
  Reshape1/1 -> Frame change2/1(V[1])  "B_i"
  [Q_oi] -> quaternion conjugate2/1
  quaternion conjugate2/1 -> Frame change2/2(Q_12)
  Propagator/2(P_TEME) -> Matrix Multiply/2
  T_JD/1 -> IGRFEmb/2(jD), Rotation matix calculation/1(T_jD)
  kep_init/1 -> Propagator/2(kep_init)

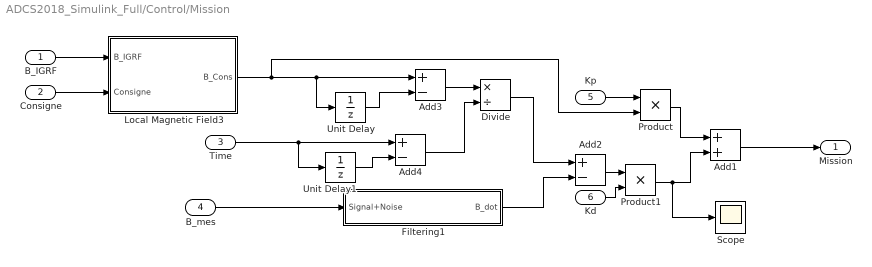
== system ADCS2018_Simulink_Full/Control/Mission ==
  B_IGRF : Inport
  Consigne : Inport  Port=2
  Time : Inport  Port=3
  B_mes : Inport  Port=4
  Kp : Inport  Port=5
  Kd : Inport  Port=6
  Add1 : Sum
  Add2 : Sum  Inputs=+-
  Add3 : Sum  Inputs=+-
  Add4 : Sum  Inputs=+-
  Divide : Product  Inputs=*/
  Filtering1 : Subsystem
  Local Magnetic Field3 : Subsystem
  Product : Product
  Product1 : Product
  Scope : Scope
  Unit Delay : UnitDelay  SampleTime=-1
  Unit Delay1 : UnitDelay  InitialCondition=-1  SampleTime=-1
  Mission : Outport
  wires:
  Add3/1 -> Divide/1
  Time/1 -> Unit Delay1/1, Add4/1
  Local Magnetic Field3/1(B_Cons) -> Product/2, Unit Delay/1, Add3/1
  Consigne/1 -> Local Magnetic Field3/2(Consigne)
  Unit Delay/1 -> Add3/2
  B_IGRF/1 -> Local Magnetic Field3/1("B_IGRF ")
  Add4/1 -> Divide/2
  Unit Delay1/1 -> Add4/2
  Product/1 -> Add1/1
  Divide/1 -> Add2/1
  B_mes/1 -> Filtering1/1(Signal+Noise)
  Add1/1 -> Mission/1
  Add2/1 -> Product1/1
  Product1/1 -> Scope/1, Add1/2
  Kd/1 -> Product1/2
  Kp/1 -> Product/1
  Filtering1/1(B_dot) -> Add2/2

== system ADCS2018_Simulink_Full/Disturbance/Gravity torque ==
  note: R_bo
  x_bo : Inport
  Demux : Demux  Outputs=7
  Gain : Gain  Gain=3*wo^2
  Inertia1 : Constant  Value=I
  Mux : Mux
  Mux1 : Mux  Inputs=3
  Product1 : Product  Multiplication=Matrix(*)
  Product2 : Product  Multiplication=Matrix(*)
  Reshape : Reshape
  Terminator : Terminator
  Variable Selector : dspindex/Variable Selector  NumInputs=1  rowsOrCols=Columns  IdxMode=Variable  Elements=[1 3]  ZerOneIdxMode=One-based  errmode=Clip Index  FillMode=on  FillValues=0
  constant : Constant  Value=3
  quat2DCM2 : Subsystem
  vect_SkewMat : My_library/vect_SkewMat
      settings: SourceProductName=My Library
  gg : Outport
  wires:
  Demux/5 -> Mux1/1
  Demux/3 -> Mux/3
  Demux/2 -> Mux/2
  Demux/4 -> Mux/4
  Mux/1 -> quat2DCM2/1(Quat)
  Demux/1 -> Mux/1
  Product2/1 -> Gain/1
  Variable Selector/1 -> vect_SkewMat/1, Product2/2
  Product1/1 -> Product2/1
  Inertia1/1 -> Product1/2
  Demux/7 -> Mux1/3
  Demux/6 -> Mux1/2
  Gain/1 -> Reshape/1
  constant/1 -> Variable Selector/2
  quat2DCM2/1(DCM) -> Variable Selector/1
  vect_SkewMat/1 -> Product1/1
  x_bo/1 -> Demux/1
  Reshape/1 -> gg/1
  Mux1/1 -> Terminator/1

== system ADCS2018_Simulink_Full/Disturbance/mag residual torque ==
  b_earth : Inport
  Cross Product : vrlib/Utilities/Cross Product
      settings: SourceProductBaseCode=VR
  residual moment : Constant  Value=mr
  mt : Outport  PortDimensions=3
  wires:
  residual moment/1 -> Cross Product/1
  Cross Product/1 -> mt/1
  b_earth/1 -> Cross Product/2

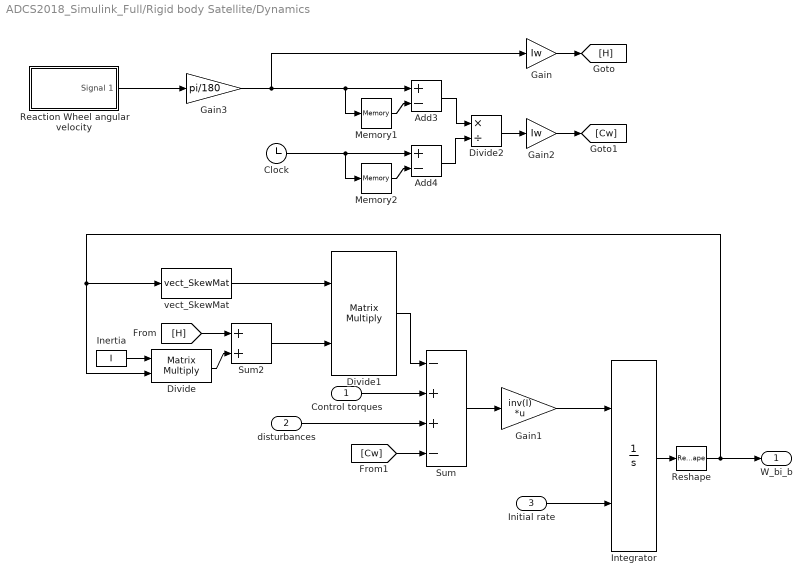
== system ADCS2018_Simulink_Full/Rigid body Satellite/Dynamics ==
  Control torques : Inport  PortDimensions=3
  disturbances : Inport  Port=2  PortDimensions=3
  Initial rate : Inport  Port=3
  Add3 : Sum  Inputs=+-
  Add4 : Sum  Inputs=+-
  Clock : Clock
  Divide : Product  Inputs=**  Multiplication=Matrix(*)
  Divide1 : Product  Inputs=**  Multiplication=Matrix(*)
  Divide2 : Product  Inputs=*/
  Gain : Gain  Gain=Iw
  Gain1 : Gain  Gain=inv(I)  Multiplication=Matrix(K*u)
  Gain2 : Gain  Gain=Iw
  Gain3 : Gain  Gain=pi/180
  Inertia : Constant  Value=I
  Integrator : Integrator  InitialConditionSource=external
  Memory1 : Memory
  Memory2 : Memory  InitialCondition=-1
  Reaction Wheel angular velocity : Subsystem  Tag=STV Subsys  LoadFcn=sigbuilder_block('load');  StartFcn=sigbuilder_block('start');  StopFcn=sigbuilder_block('stop');  ClipboardFcn=sigbuilder_block('clipboard');  mask(Sigbuilder block){tuvar=[0:10]}
      mask help: Simulink:masks:SigbuilderBlock_MD
      mask init:
      | if ~strcmp(get_param(bdroot(gcbh),'SimulationStatus'),'stopped') tuvar = sigbuilder_block('maskInit'); end
      settings: CopyFcn=sigbuilder_block('copy');  DeleteFcn=sigbuilder_block('delete');  ModelCloseFcn=sigbuilder_block('modelClose');  PreSaveFcn=sigbuilder_block('preSave');  PauseFcn=sigbuilder_block('pause');  ContinueFcn=sigbuilder_block('continue');  NameChangeFcn=sigbuilder_block('namechange');  OpenFcn=sigbuilder_block('open',[217.5 258 1141.5 361.5 ]);  CloseFcn=sigbuilder_block('close');
      mask Display: plot(0, 0, 100, 100,[2, 2, 32, 32, 2], [68, 8, 8, 68, 68],[32, 2], [38, 38], [32, 19, 2],[53, 60, 44], [32, 17, 17, 2],[16, 16, 31, 31]);txt = getActiveGroup(gcbh);text(2, 100, txt,'verticalAlignment', 'top');
  Reshape : Reshape
  Sum : Sum  Inputs=-++-
  Sum2 : Sum
  vect_SkewMat : My_library/vect_SkewMat
      settings: SourceProductName=My Library
  W_bi_b : Outport
  wires:
  disturbances/1 -> Sum/3
  Control torques/1 -> Sum/2
  Integrator/1 -> Reshape/1
  Sum/1 -> Gain1/1
  Divide1/1 -> Sum/1
  Gain1/1 -> Integrator/1
  Initial rate/1 -> Integrator/2
  Reshape/1 -> vect_SkewMat/1, Divide/2, W_bi_b/1
  Inertia/1 -> Divide/1
  Divide/1 -> Sum2/2
  vect_SkewMat/1 -> Divide1/1
  Sum2/1 -> Divide1/2
  [H] -> Sum2/1
  [Cw] -> Sum/4
  Gain/1 -> [H]
  Gain2/1 -> [Cw]
  Memory1/1 -> Add3/2
  Memory2/1 -> Add4/2
  Add3/1 -> Divide2/1
  Add4/1 -> Divide2/2
  Gain3/1 -> Add3/1, Memory1/1, Gain/1
  Clock/1 -> Memory2/1, Add4/1
  Reaction Wheel angular velocity/1(Signal 1) -> Gain3/1
  Divide2/1 -> Gain2/1

== system ADCS2018_Simulink_Full/Rigid body Satellite/Kinematics ==
  W_bi_b : Inport
  Init quat : Inport  Port=2
  Constant : Constant  Value=0
  Integrator : Integrator  InitialConditionSource=external
  Mux : Mux  Inputs=2
  Product : Product  Multiplication=Matrix(*)
  quatSkew : Subsystem
  quat_normalise : My_library/quat_normalise
      settings: SourceProductName=My Library
  w_mat1 : Gain  Gain=1/2
  Q_bi : Outport
  wires:
  Integrator/1 -> quat_normalise/1
  W_bi_b/1 -> Mux/2
  Mux/1 -> Product/2
  quatSkew/1(quat skew) -> Product/1
  w_mat1/1 -> quatSkew/1(quat)
  Init quat/1 -> Integrator/2
  Product/1 -> Integrator/1
  quat_normalise/1 -> w_mat1/1, Q_bi/1
  Constant/1 -> Mux/1

== system ADCS2018_Simulink_Full/Simulation IGRF/Rotation matix calculation ==
  T_jD : Inport
  Constant : Constant  Value=0
  Constant1 : Constant
  GMST calculation : Subsystem
  Gain2 : Gain  Gain=-1
  Matrix Concatenate : Concatenate  NumInputs=3  Mode=Multidimensional array  ConcatenateDimension=2
  Mux : Mux  Inputs=3
  Mux2 : Mux  Inputs=3
  Mux3 : Mux  Inputs=3
  Reshape : Reshape
  Reshape1 : Reshape
  Reshape2 : Reshape
  sincos : Trigonometry  Operator=sincos
  M_TEMEECEF : Outport
  wires:
  Mux2/1 -> Reshape1/1
  Mux/1 -> Reshape/1
  Reshape1/1 -> Matrix Concatenate/2
  Mux3/1 -> Reshape2/1
  Reshape/1 -> Matrix Concatenate/1
  Reshape2/1 -> Matrix Concatenate/3
  Constant/1 -> Mux3/1, Mux3/2, Mux/3, Mux2/3
  Constant1/1 -> Mux3/3
  sincos/2 -> Mux2/2, Mux/1
  Matrix Concatenate/1 -> M_TEMEECEF/1
  sincos/1 -> Mux2/1, Gain2/1
  T_jD/1 -> GMST calculation/1(T_jD)
  GMST calculation/1(GMST) -> sincos/1
  Gain2/1 -> Mux/2

== system ADCS2018_Simulink_Full/Control/IGRF on bord/Frame change2 ==
  V[1] : Inport
  Q_12 : Inport  Port=2
  Constant7 : Constant  Value=0
  Demux1 : Demux
  Mux6 : Mux  Inputs=2
  Mux7 : Mux  Inputs=3
  Terminator2 : Terminator
  q : InportShadow  Port=2
  quat multiply4 : My_library/quat multiply
      settings: SourceProductName=My Library
  quat multiply5 : My_library/quat multiply
      settings: SourceProductName=My Library
  quaternion conjugate2 : My_library/quaternion conjugate
      settings: SourceProductName=My Library
  "V[2] " : Outport
  wires:
  Demux1/4 -> Mux7/3
  Q_12/1 -> quat multiply4/1
  quat multiply5/1 -> Demux1/1
  quat multiply4/1 -> quat multiply5/1
  Mux6/1 -> quat multiply4/2
  Demux1/2 -> Mux7/1
  Demux1/1 -> Terminator2/1
  q/1 -> quaternion conjugate2/1
  quaternion conjugate2/1 -> quat multiply5/2
  Demux1/3 -> Mux7/2
  Constant7/1 -> Mux6/1
  Mux7/1 -> "V[2] "/1  "x_b_o"
  V[1]/1 -> Mux6/2

== system ADCS2018_Simulink_Full/Control/IGRF on bord/Rotation matix calculation ==
  T_jD : Inport
  Constant : Constant  Value=0
  Constant1 : Constant
  GMST calculation : Subsystem
  Gain2 : Gain  Gain=-1
  Matrix Concatenate : Concatenate  NumInputs=3  Mode=Multidimensional array  ConcatenateDimension=2
  Mux : Mux  Inputs=3
  Mux2 : Mux  Inputs=3
  Mux3 : Mux  Inputs=3
  Reshape : Reshape
  Reshape1 : Reshape
  Reshape2 : Reshape
  sincos : Trigonometry  Operator=sincos
  M_TEMEECEF : Outport
  wires:
  Mux2/1 -> Reshape1/1
  Mux/1 -> Reshape/1
  Reshape1/1 -> Matrix Concatenate/2
  Mux3/1 -> Reshape2/1
  Reshape/1 -> Matrix Concatenate/1
  Reshape2/1 -> Matrix Concatenate/3
  Constant/1 -> Mux3/1, Mux3/2, Mux/3, Mux2/3
  Constant1/1 -> Mux3/3
  sincos/2 -> Mux2/2, Mux/1
  Matrix Concatenate/1 -> M_TEMEECEF/1
  sincos/1 -> Mux2/1, Gain2/1
  T_jD/1 -> GMST calculation/1(T_jD)
  GMST calculation/1(GMST) -> sincos/1
  Gain2/1 -> Mux/2

== system ADCS2018_Simulink_Full/Control/Mission/Filtering1 ==
  Signal+Noise : Inport
  -a1 : Gain  Gain=-a1
  Add2 : Sum  Inputs=|++
  Add3 : Sum
  Unit Delay : UnitDelay  SampleTime=-1
  Unit Delay1 : UnitDelay  SampleTime=-1
  b0 : Gain  Gain=b0
  b1 : Gain  Gain=b1
  B_dot : Outport
  wires:
  Add2/1 -> Unit Delay1/1, B_dot/1
  b0/1 -> Add2/1
  Signal+Noise/1 -> b0/1, Unit Delay/1
  b1/1 -> Add3/1
  Unit Delay/1 -> b1/1
  -a1/1 -> Add3/2
  Unit Delay1/1 -> -a1/1
  Add3/1 -> Add2/2

== system ADCS2018_Simulink_Full/Control/Mission/Local Magnetic Field3 ==
  "B_IGRF " : Inport  PortDimensions=3
  Consigne : Inport  Port=2
  Demux1 : Demux  Outputs=7
  Frame change2 : Subsystem
  Mux : Mux
  Mux5 : Mux  Inputs=3
  No need for the angular velocity : Terminator
  B_Cons : Outport  PortDimensions=3
  wires:
  Consigne/1 -> Demux1/1
  Demux1/5 -> Mux5/1
  Demux1/6 -> Mux5/2
  Demux1/7 -> Mux5/3
  Mux5/1 -> No need for the angular velocity/1
  Mux/1 -> Frame change2/2(Q_12)
  Demux1/1 -> Mux/1
  Demux1/2 -> Mux/2
  Demux1/3 -> Mux/3
  Demux1/4 -> Mux/4
  "B_IGRF "/1 -> Frame change2/1(V[1])
  Frame change2/1("V[2] ") -> B_Cons/1

== system ADCS2018_Simulink_Full/Disturbance/Gravity torque/quat2DCM2 ==
  Quat : Inport  PortDimensions=4
  Subsystem : Subsystem
  Subsystem1 : Subsystem
  Subsystem2 : Subsystem
  Subsystem3 : Subsystem
  Subsystem4 : Subsystem
  Subsystem5 : Subsystem
  Subsystem6 : Subsystem
  Subsystem7 : Subsystem
  Subsystem8 : Subsystem
  Subsystem9 : Subsystem
  quat_normalise : My_library/quat_normalise
      settings: SourceProductName=My Library
  DCM : Outport  PortDimensions=[3,3]  InitialOutput=0
  wires:
  Subsystem/1(Matrix) -> DCM/1
  Subsystem1/1(A11) -> Subsystem/1(M11)
  Subsystem4/1(A21) -> Subsystem/4(M21)
  Subsystem7/1(A31) -> Subsystem/7(M31)
  Subsystem8/1(A32) -> Subsystem/8(M32)
  Subsystem9/1(A33) -> Subsystem/9(M33)
  Quat/1 -> quat_normalise/1
  quat_normalise/1 -> Subsystem1/1(normal(q)), Subsystem2/1(normal(q)), Subsystem3/1(normal(q)), Subsystem4/1(normal(q)), Subsystem5/1(normal(q)), Subsystem6/1(normal(q)), Subsystem7/1(normal(q)), Subsystem9/1(normal(q)), Subsystem8/1(normal(q))
  Subsystem5/1(A22) -> Subsystem/5(M22)
  Subsystem2/1(A12) -> Subsystem/2(M12)
  Subsystem3/1(A13) -> Subsystem/3(M13)
  Subsystem6/1(A23) -> Subsystem/6(M23)

== system ADCS2018_Simulink_Full/Rigid body Satellite/Dynamics/Reaction Wheel angular velocity ==
  Demux : Demux  Tag=STV Demux  Outputs=1
  FromWs : FromWorkspace  Tag=STV FromWs  VariableName=tuvar  SampleTime=0
      SigBuilderData=|
      | common.afterFinalStr = 'Extrapolate'
      | common.sampleTime = 0
      | dataSet.timeRange = [0 146369.116664]
      | dataSet.name = 'Group 1'
      | sbobj.Groups.Name = 'Group 1'
      | sbobj.Groups.Signals.Name = 'Signal 1'
      | sbobj.Groups.Signals.XData = [0 20000 30000 146369.116664]
      | sbobj.Groups.Signals.YData = [0 0 8000 8000]
      | sbobj.Groups.TimeRange = [0 146369.116664]
  Signal 1 : Outport  Tag=STV Outport
  wires:
  Demux/1 -> Signal 1/1
  FromWs/1 -> Demux/1

== system ADCS2018_Simulink_Full/Rigid body Satellite/Kinematics/quatSkew ==
  quat : Inport
  Demux1 : Demux
  Gain1 : Gain  Gain=-1
  Gain2 : Gain  Gain=-1
  Gain3 : Gain  Gain=-1
  Matrix Concatenate : Concatenate  NumInputs=4  Mode=Multidimensional array  ConcatenateDimension=2
  Mux{,1..3} (4 alike) : Mux
  Reshape{,1..3} (4 alike) : Reshape
  quat skew : Outport
  wires:
  Reshape/1 -> Matrix Concatenate/1
  Mux2/1 -> Reshape2/1
  Mux/1 -> Reshape/1
  quat/1 -> Demux1/1
  Matrix Concatenate/1 -> quat skew/1
  Mux1/1 -> Reshape1/1
  Reshape1/1 -> Matrix Concatenate/2
  Reshape2/1 -> Matrix Concatenate/3
  Reshape3/1 -> Matrix Concatenate/4
  Mux3/1 -> Reshape3/1
  Demux1/4 -> Gain3/1, Mux1/3, Mux/4
  Demux1/3 -> Gain2/1, Mux3/2, Mux/3
  Demux1/2 -> Gain1/1, Mux2/4, Mux/2
  Demux1/1 -> Mux3/4, Mux2/3, Mux1/2, Mux/1
  Gain1/1 -> Mux3/3, Mux1/1
  Gain2/1 -> Mux2/1, Mux1/4
  Gain3/1 -> Mux3/1, Mux2/2

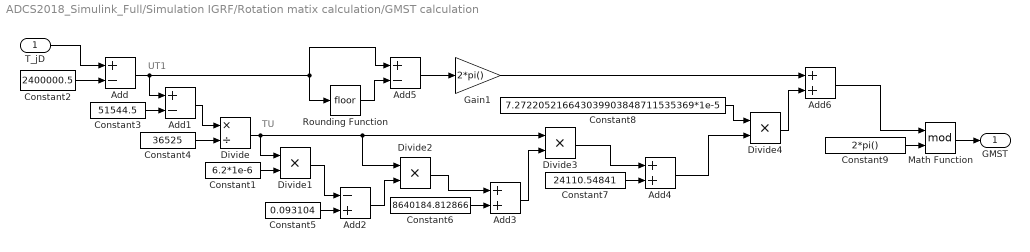
== system ADCS2018_Simulink_Full/Simulation IGRF/Rotation matix calculation/GMST calculation ==
  note: TU
  note: UT1
  T_jD : Inport
  Add : Sum  Inputs=+-
  Add1 : Sum  Inputs=+-
  Add2 : Sum  Inputs=-+
  Add3 : Sum
  Add4 : Sum
  Add5 : Sum  Inputs=+-
  Add6 : Sum
  Constant1 : Constant  Value=6.2*1e-6
  Constant2 : Constant  Value=2400000.5
  Constant3 : Constant  Value=51544.5
  Constant4 : Constant  Value=36525
  Constant5 : Constant  Value=0.093104
  Constant6 : Constant  Value=8640184.812866
  Constant7 : Constant  Value=24110.54841
  Constant8 : Constant  Value=7.272205216643039903848711535369*1e-5
  Constant9 : Constant  Value=2*pi()
  Divide : Product  Inputs=*/
  Divide{1..4} (4 alike) : Product  Inputs=**
  Gain1 : Gain  Gain=2*pi()
  Math Function : Math  Operator=mod  SaturateOnIntegerOverflow=on
  Rounding Function : Rounding
  GMST : Outport
  wires:
  Divide2/1 -> Add3/1
  Add6/1 -> Math Function/1
  Math Function/1 -> GMST/1
  Add5/1 -> Gain1/1
  Constant6/1 -> Add3/2
  Constant3/1 -> Add1/2
  Add2/1 -> Divide2/2
  Constant7/1 -> Add4/2
  Add1/1 -> Divide/1
  Gain1/1 -> Add6/1
  Constant8/1 -> Divide4/1
  Divide4/1 -> Add6/2
  Add3/1 -> Divide3/2
  Constant2/1 -> Add/2
  Add/1 -> Add1/1, Rounding Function/1, Add5/1
  Constant9/1 -> Math Function/2
  Add4/1 -> Divide4/2
  Rounding Function/1 -> Add5/2
  Divide/1 -> Divide1/1, Divide3/1, Divide2/1
  Constant1/1 -> Divide1/2
  Constant4/1 -> Divide/2
  T_jD/1 -> Add/1
  Constant5/1 -> Add2/2
  Divide1/1 -> Add2/1
  Divide3/1 -> Add4/1

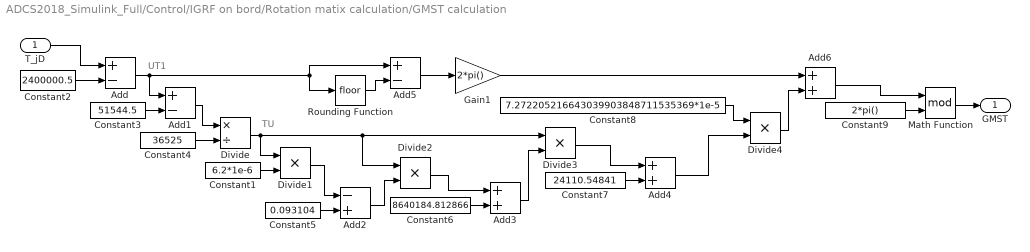
== system ADCS2018_Simulink_Full/Control/IGRF on bord/Rotation matix calculation/GMST calculation ==
  note: TU
  note: UT1
  T_jD : Inport
  Add : Sum  Inputs=+-
  Add1 : Sum  Inputs=+-
  Add2 : Sum  Inputs=-+
  Add3 : Sum
  Add4 : Sum
  Add5 : Sum  Inputs=+-
  Add6 : Sum
  Constant1 : Constant  Value=6.2*1e-6
  Constant2 : Constant  Value=2400000.5
  Constant3 : Constant  Value=51544.5
  Constant4 : Constant  Value=36525
  Constant5 : Constant  Value=0.093104
  Constant6 : Constant  Value=8640184.812866
  Constant7 : Constant  Value=24110.54841
  Constant8 : Constant  Value=7.272205216643039903848711535369*1e-5
  Constant9 : Constant  Value=2*pi()
  Divide : Product  Inputs=*/
  Divide{1..4} (4 alike) : Product  Inputs=**
  Gain1 : Gain  Gain=2*pi()
  Math Function : Math  Operator=mod  SaturateOnIntegerOverflow=on
  Rounding Function : Rounding
  GMST : Outport
  wires:
  Divide2/1 -> Add3/1
  Add6/1 -> Math Function/1
  Math Function/1 -> GMST/1
  Add5/1 -> Gain1/1
  Constant6/1 -> Add3/2
  Constant3/1 -> Add1/2
  Add2/1 -> Divide2/2
  Constant7/1 -> Add4/2
  Add1/1 -> Divide/1
  Gain1/1 -> Add6/1
  Constant8/1 -> Divide4/1
  Divide4/1 -> Add6/2
  Add3/1 -> Divide3/2
  Constant2/1 -> Add/2
  Add/1 -> Add1/1, Rounding Function/1, Add5/1
  Constant9/1 -> Math Function/2
  Add4/1 -> Divide4/2
  Rounding Function/1 -> Add5/2
  Divide/1 -> Divide1/1, Divide3/1, Divide2/1
  Constant1/1 -> Divide1/2
  Constant4/1 -> Divide/2
  T_jD/1 -> Add/1
  Constant5/1 -> Add2/2
  Divide1/1 -> Add2/1
  Divide3/1 -> Add4/1

== system ADCS2018_Simulink_Full/Control/Mission/Local Magnetic Field3/Frame change2 ==
  V[1] : Inport
  Q_12 : Inport  Port=2
  Constant7 : Constant  Value=0
  Demux1 : Demux
  Mux6 : Mux  Inputs=2
  Mux7 : Mux  Inputs=3
  Terminator2 : Terminator
  q : InportShadow  Port=2
  quat multiply4 : My_library/quat multiply
      settings: SourceProductName=My Library
  quat multiply5 : My_library/quat multiply
      settings: SourceProductName=My Library
  quaternion conjugate2 : My_library/quaternion conjugate
      settings: SourceProductName=My Library
  "V[2] " : Outport
  wires:
  Demux1/4 -> Mux7/3
  Q_12/1 -> quat multiply4/1
  quat multiply5/1 -> Demux1/1
  quat multiply4/1 -> quat multiply5/1
  Mux6/1 -> quat multiply4/2
  Demux1/2 -> Mux7/1
  Demux1/1 -> Terminator2/1
  q/1 -> quaternion conjugate2/1
  quaternion conjugate2/1 -> quat multiply5/2
  Demux1/3 -> Mux7/2
  Constant7/1 -> Mux6/1
  Mux7/1 -> "V[2] "/1  "x_b_o"
  V[1]/1 -> Mux6/2

== system ADCS2018_Simulink_Full/Disturbance/Gravity torque/quat2DCM2/Subsystem ==
  M11 : Inport  PortDimensions=1
  M12 : Inport  Port=2  PortDimensions=1
  M13 : Inport  Port=3  PortDimensions=1
  M21 : Inport  Port=4  PortDimensions=1
  M22 : Inport  Port=5  PortDimensions=1
  M23 : Inport  Port=6  PortDimensions=1
  M31 : Inport  Port=7  PortDimensions=1
  M32 : Inport  Port=8  PortDimensions=1
  M33 : Inport  Port=9  PortDimensions=1
  Reshape (9) to [3x3] column-major : Reshape  OutputDimensionality=Customize  OutputDimensions=[3,3]
  Vector Concatenate : Concatenate  NumInputs=9
  Matrix : Outport  PortDimensions=[3 3]
  wires:
  M32/1 -> Vector Concatenate/6
  M13/1 -> Vector Concatenate/7
  M33/1 -> Vector Concatenate/9
  M23/1 -> Vector Concatenate/8
  M11/1 -> Vector Concatenate/1
  Vector Concatenate/1 -> Reshape (9) to [3x3] column-major/1
  M21/1 -> Vector Concatenate/2
  M22/1 -> Vector Concatenate/5
  M31/1 -> Vector Concatenate/3
  M12/1 -> Vector Concatenate/4
  Reshape (9) to [3x3] column-major/1 -> Matrix/1

== system ADCS2018_Simulink_Full/Disturbance/Gravity torque/quat2DCM2/Subsystem1 ==
  normal(q) : Inport
  Demux : Demux
  Product{,1..3} (4 alike) : Product  RndMeth=Zero
  Sum : Sum  Inputs=++--
  A11 : Outport
  wires:
  Demux/2 -> Product2/1, Product2/2
  Product2/1 -> Sum/2
  Product3/1 -> Sum/1
  Product/1 -> Sum/4
  Product1/1 -> Sum/3
  Sum/1 -> A11/1
  Demux/3 -> Product1/1, Product1/2
  normal(q)/1 -> Demux/1
  Demux/1 -> Product3/1, Product3/2
  Demux/4 -> Product/1, Product/2

== system ADCS2018_Simulink_Full/Disturbance/Gravity torque/quat2DCM2/Subsystem2 ==
  normal(q) : Inport
  Demux : Demux
  Gain : Gain  Gain=2
  Product2 : Product  RndMeth=Zero
  Product3 : Product  RndMeth=Zero
  Sum : Sum  Inputs=|++
  A12 : Outport
  wires:
  Sum/1 -> Gain/1
  normal(q)/1 -> Demux/1
  Gain/1 -> A12/1
  Product2/1 -> Sum/2
  Demux/1 -> Product3/2
  Product3/1 -> Sum/1
  Demux/4 -> Product3/1
  Demux/2 -> Product2/1
  Demux/3 -> Product2/2

== system ADCS2018_Simulink_Full/Disturbance/Gravity torque/quat2DCM2/Subsystem3 ==
  normal(q) : Inport
  Demux : Demux
  Gain : Gain  Gain=2
  Product1 : Product  RndMeth=Zero
  Product2 : Product  RndMeth=Zero
  Sum : Sum  Inputs=|-+
  A13 : Outport
  wires:
  Demux/2 -> Product2/1
  Gain/1 -> A13/1
  Product2/1 -> Sum/2
  normal(q)/1 -> Demux/1
  Demux/3 -> Product1/2
  Product1/1 -> Sum/1
  Sum/1 -> Gain/1
  Demux/4 -> Product2/2
  Demux/1 -> Product1/1

== system ADCS2018_Simulink_Full/Disturbance/Gravity torque/quat2DCM2/Subsystem4 ==
  normal(q) : Inport
  Demux : Demux
  Gain : Gain  Gain=2
  Product2 : Product  RndMeth=Zero
  Product3 : Product  RndMeth=Zero
  Sum : Sum  Inputs=|-+
  A21 : Outport
  wires:
  Product2/1 -> Sum/2
  normal(q)/1 -> Demux/1
  Product3/1 -> Sum/1
  Sum/1 -> Gain/1
  Demux/3 -> Product2/2
  Demux/4 -> Product3/1
  Demux/1 -> Product3/2
  Gain/1 -> A21/1
  Demux/2 -> Product2/1

== system ADCS2018_Simulink_Full/Disturbance/Gravity torque/quat2DCM2/Subsystem5 ==
  normal(q) : Inport
  Demux : Demux
  Product{,1..3} (4 alike) : Product  RndMeth=Zero
  Sum : Sum  Inputs=+-+-
  A22 : Outport
  wires:
  Demux/2 -> Product2/2, Product2/1
  Sum/1 -> A22/1
  Product2/1 -> Sum/2
  Product1/1 -> Sum/3
  Demux/3 -> Product1/2, Product1/1
  Demux/4 -> Product/2, Product/1
  Demux/1 -> Product3/2, Product3/1
  Product3/1 -> Sum/1
  Product/1 -> Sum/4
  normal(q)/1 -> Demux/1

== system ADCS2018_Simulink_Full/Disturbance/Gravity torque/quat2DCM2/Subsystem6 ==
  normal(q) : Inport
  Demux : Demux
  Gain : Gain  Gain=2
  Product1 : Product  RndMeth=Zero
  Product2 : Product  RndMeth=Zero
  Sum : Sum  Inputs=|++
  A23 : Outport
  wires:
  Gain/1 -> A23/1
  Product2/1 -> Sum/2
  Sum/1 -> Gain/1
  Demux/2 -> Product1/2
  Demux/4 -> Product2/2
  normal(q)/1 -> Demux/1
  Product1/1 -> Sum/1
  Demux/1 -> Product1/1
  Demux/3 -> Product2/1

== system ADCS2018_Simulink_Full/Disturbance/Gravity torque/quat2DCM2/Subsystem7 ==
  normal(q) : Inport
  Demux : Demux
  Gain : Gain  Gain=2
  Product1 : Product  RndMeth=Zero
  Product2 : Product  RndMeth=Zero
  Sum : Sum  Inputs=|++
  A31 : Outport
  wires:
  Demux/3 -> Product1/2
  Demux/1 -> Product1/1
  Product1/1 -> Sum/1
  Sum/1 -> Gain/1
  normal(q)/1 -> Demux/1
  Product2/1 -> Sum/2
  Demux/2 -> Product2/1
  Demux/4 -> Product2/2
  Gain/1 -> A31/1

== system ADCS2018_Simulink_Full/Disturbance/Gravity torque/quat2DCM2/Subsystem8 ==
  normal(q) : Inport
  Demux : Demux
  Gain : Gain  Gain=2
  Product1 : Product  RndMeth=Zero
  Product2 : Product  RndMeth=Zero
  Sum : Sum  Inputs=|-+
  A32 : Outport
  wires:
  Product1/1 -> Sum/1
  Sum/1 -> Gain/1
  Gain/1 -> A32/1
  Demux/3 -> Product2/1
  Demux/4 -> Product2/2
  Product2/1 -> Sum/2
  normal(q)/1 -> Demux/1
  Demux/2 -> Product1/2
  Demux/1 -> Product1/1

== system ADCS2018_Simulink_Full/Disturbance/Gravity torque/quat2DCM2/Subsystem9 ==
  normal(q) : Inport
  Demux : Demux
  Product{,1..3} (4 alike) : Product  RndMeth=Zero
  Sum : Sum  Inputs=+--+
  A33 : Outport
  wires:
  Product3/1 -> Sum/1
  Product/1 -> Sum/4
  Demux/3 -> Product1/2, Product1/1
  Product2/1 -> Sum/2
  Product1/1 -> Sum/3
  Sum/1 -> A33/1
  Demux/1 -> Product3/2, Product3/1
  Demux/4 -> Product/2, Product/1
  normal(q)/1 -> Demux/1
  Demux/2 -> Product2/2, Product2/1

== matlab function ADCS2018_Simulink_Full/speed cal/MATLAB Function ==
  settings: updateMethod=DISCRETE
  data: u input; y output
function y = fcn(u)
%#codegen
coder.extrinsic('clock','etime')
y=0;
persistent tin

if isempty(tin)
tin=clock;
end

tnow = clock;
tsecs=etime(tnow,tin);

y=u/tsecs;

== matlab function ADCS2018_Simulink_Full/MATLAB Function ==
  data: t input; T_JD output; tinit input
function T_JD = fcn(t, tinit)
%#codegen
tinit(6)=tinit(6)+t;
T_JD=Dt2jD(tinit);
